simulink model "nn_fuel_control_4_10"  (R2021a)
settings: Solver=ode15s  StartTime=0.0  StopTime=T  MaxStep=.01  RelTol=1e-3
undefined symbols (not defined in the file): AF_sensor_tol, fault_time, fuel_inj_tol, kappa_tol, MAF_sensor_tol, pump_tol, tau_ww_tol
libraries: neural x46
(part 2 of 2)

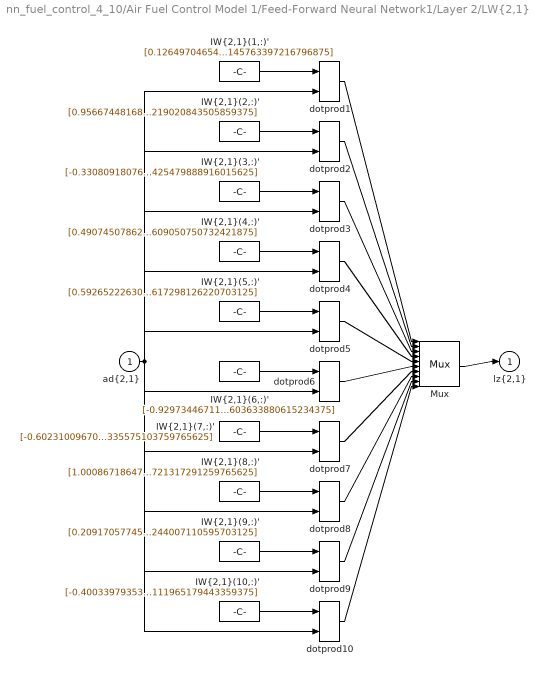
== system nn_fuel_control_4_10/Air Fuel Control Model 1/Feed-Forward Neural Network1/Layer 2/LW{2,1} ==
  "ad{2,1}" : Inport  PortDimensions=10
      mask Display: e = 0.06;c1 = [120 230 180]/255;c2 = ([120 230 180]+0)/(256+128);c3 = ([120 230 180]+128)/(256+128);patch([0 1 1 0],[0 0 1 1],c1);patch([0 1 1 1-e 1-e 0+e],[0 0 1 1-e 0+e 0+e],c2);patch([0 0 1 1-e 0+e 0+e],[0 1 1 1-e 1-e 0+e],c3);plot([0 1 1 0 0],[0 0 1 1 0]);
  "IW{2,1}(1,:)'" : Constant  Value=[0.126497046544859215178036038196296431124210357666015625;0.75221409398679295321699100895784795284271240234375;-0.1950995321727321540894450890846201218664646148681640625;-0.76593928444443459824242381728254258632659912109375;0.06664328726876174446847045373942819423973560333251953125;-0.21742718572034547275251270548324100673198699951171875;1.0030759253859538038256005165749229490756988525390625;-0.7869649700269818470843574687023647129535675048828125;0.556124501951611449612755677662789821624755859375;-0.52293583386677500168815413417178206145763397216796875]
      mask Display: e = 0.06;c1 = [120 150 230]/255;c2 = ([120 150 230]+0)/383;c3 = ([120 150 230]+128)/383;patch([0 1 1 0],[0 0 1 1],c1);patch([0 1 1 1-e 1-e 0+e],[0 0 1 1-e 0+e 0+e],c2);patch([0 0 1 1-e 0+e 0+e],[0 1 1 1-e 1-e 0+e],c3);plot([0 1 1 0 0],[0 0 1 1 0]);disp('weights');
  "IW{2,1}(10,:)'" : Constant  Value=[-0.4003397935387604800183680708869360387325286865234375;-0.9760537487034819381648276248597539961338043212890625;-0.661362482630752257506401292630471289157867431640625;-0.5845508787619853041661599490907974541187286376953125;0.7079823054105311985750859093968756496906280517578125;0.87748572874551289402234033332206308841705322265625;-0.530069953204840516036711051128804683685302734375;-0.848837519709181531624153649318031966686248779296875;-0.9175382615241487460622238359064795076847076416015625;0.27264837844771871999682844034396111965179443359375]
      mask Display: e = 0.06;c1 = [120 150 230]/255;c2 = ([120 150 230]+0)/383;c3 = ([120 150 230]+128)/383;patch([0 1 1 0],[0 0 1 1],c1);patch([0 1 1 1-e 1-e 0+e],[0 0 1 1-e 0+e 0+e],c2);patch([0 0 1 1-e 0+e 0+e],[0 1 1 1-e 1-e 0+e],c3);plot([0 1 1 0 0],[0 0 1 1 0]);disp('weights');
  "IW{2,1}(2,:)'" : Constant  Value=[0.95667448168226798532742805036832578480243682861328125;0.85004275325366618343281288616708479821681976318359375;0.359542314700540099892123180325143039226531982421875;-0.6107936641860096660394674472627229988574981689453125;-0.031298787731731524119904719327678321860730648040771484375;-0.52979378096300411282726372519391588866710662841796875;-0.567955949619257438598651788197457790374755859375;-0.12292161961932319969026394801403512246906757354736328125;0.236880433739087070676987423212267458438873291015625;-0.50914689409082070081780102555057965219020843505859375]
      mask Display: e = 0.06;c1 = [120 150 230]/255;c2 = ([120 150 230]+0)/383;c3 = ([120 150 230]+128)/383;patch([0 1 1 0],[0 0 1 1],c1);patch([0 1 1 1-e 1-e 0+e],[0 0 1 1-e 0+e 0+e],c2);patch([0 0 1 1-e 0+e 0+e],[0 1 1 1-e 1-e 0+e],c3);plot([0 1 1 0 0],[0 0 1 1 0]);disp('weights');
  "IW{2,1}(3,:)'" : Constant  Value=[-0.33080918076060328303356072865426540374755859375;-0.91079242740214727547254369710572063922882080078125;-0.7216409660489764288371361544704996049404144287109375;0.40560109332833160777909142780117690563201904296875;0.7487410521856288081465891082189045846462249755859375;-0.1792937276454249495571957595529966056346893310546875;-0.7489244995021773210197579828673042356967926025390625;-0.950832663107312736627818594570271670818328857421875;-0.98403189361767484655274529359303414821624755859375;-0.594933336252129407739630551077425479888916015625]
      mask Display: e = 0.06;c1 = [120 150 230]/255;c2 = ([120 150 230]+0)/383;c3 = ([120 150 230]+128)/383;patch([0 1 1 0],[0 0 1 1],c1);patch([0 1 1 1-e 1-e 0+e],[0 0 1 1-e 0+e 0+e],c2);patch([0 0 1 1-e 0+e 0+e],[0 1 1 1-e 1-e 0+e],c3);plot([0 1 1 0 0],[0 0 1 1 0]);disp('weights');
  "IW{2,1}(4,:)'" : Constant  Value=[0.490745078629539699388573126270784996449947357177734375;0.669675741776368571578359478735364973545074462890625;-0.7389705859394559706032623580540530383586883544921875;-0.32518846889059016547207647818140685558319091796875;0.7292180816896500772372746723704040050506591796875;0.40551505484997385497791810848866589367389678955078125;-0.8624031920599921630099515823530964553356170654296875;0.406935627679185174532250357515295036137104034423828125;0.82694047359766609250897317906492389738559722900390625;-0.828463743887304371327218177611939609050750732421875]
      mask Display: e = 0.06;c1 = [120 150 230]/255;c2 = ([120 150 230]+0)/383;c3 = ([120 150 230]+128)/383;patch([0 1 1 0],[0 0 1 1],c1);patch([0 1 1 1-e 1-e 0+e],[0 0 1 1-e 0+e 0+e],c2);patch([0 0 1 1-e 0+e 0+e],[0 1 1 1-e 1-e 0+e],c3);plot([0 1 1 0 0],[0 0 1 1 0]);disp('weights');
  "IW{2,1}(5,:)'" : Constant  Value=[0.59265222630545533188950457770260982215404510498046875;0.6513005697610807498421081618289463222026824951171875;0.832729947816391646853162455954588949680328369140625;-0.499949414926917246049242748995311558246612548828125;0.15275099522523305495269596576690673828125;-0.2200642403627948995303853507721214555203914642333984375;0.29279576118233363590803719489485956728458404541015625;0.967351346440282977567903799354098737239837646484375;0.4551810898529715654348137832130305469036102294921875;-0.19101879400775001460743851566803641617298126220703125]
      mask Display: e = 0.06;c1 = [120 150 230]/255;c2 = ([120 150 230]+0)/383;c3 = ([120 150 230]+128)/383;patch([0 1 1 0],[0 0 1 1],c1);patch([0 1 1 1-e 1-e 0+e],[0 0 1 1-e 0+e 0+e],c2);patch([0 0 1 1-e 0+e 0+e],[0 1 1 1-e 1-e 0+e],c3);plot([0 1 1 0 0],[0 0 1 1 0]);disp('weights');
  "IW{2,1}(6,:)'" : Constant  Value=[-0.929734467111477780321138197905384004116058349609375;-0.20633861665115471595299823093228042125701904296875;0.243861218275130742227929658838547766208648681640625;-0.1569894136270153506274027677136473357677459716796875;-0.1436763750970591058120362504268996417522430419921875;-0.721299534939905395702908208477310836315155029296875;-0.8723462156088059860081784790963865816593170166015625;-0.7906932906879029498981026335968635976314544677734375;-0.2135932946365211027028863099985755980014801025390625;0.625957171841073911622288505895994603633880615234375]
      mask Display: e = 0.06;c1 = [120 150 230]/255;c2 = ([120 150 230]+0)/383;c3 = ([120 150 230]+128)/383;patch([0 1 1 0],[0 0 1 1],c1);patch([0 1 1 1-e 1-e 0+e],[0 0 1 1-e 0+e 0+e],c2);patch([0 0 1 1-e 0+e 0+e],[0 1 1 1-e 1-e 0+e],c3);plot([0 1 1 0 0],[0 0 1 1 0]);disp('weights');
  "IW{2,1}(7,:)'" : Constant  Value=[-0.602310096703943198548358850530348718166351318359375;0.73376329364989967274368609650991857051849365234375;0.95498454377033947793051993357948958873748779296875;0.9141420095755534713788392764399759471416473388671875;-0.99757823216680474587292337673716247081756591796875;0.388190532974689528344924838165752589702606201171875;0.232893122124527618410638751811347901821136474609375;0.4600844221479103435257229648414067924022674560546875;-0.4005592463439544559378191479481756687164306640625;-0.4404459192897596242488589268759824335575103759765625]
      mask Display: e = 0.06;c1 = [120 150 230]/255;c2 = ([120 150 230]+0)/383;c3 = ([120 150 230]+128)/383;patch([0 1 1 0],[0 0 1 1],c1);patch([0 1 1 1-e 1-e 0+e],[0 0 1 1-e 0+e 0+e],c2);patch([0 0 1 1-e 0+e 0+e],[0 1 1 1-e 1-e 0+e],c3);plot([0 1 1 0 0],[0 0 1 1 0]);disp('weights');
  "IW{2,1}(8,:)'" : Constant  Value=[1.0008671864742602064524135130341164767742156982421875;0.627994547262577640367453568615019321441650390625;-0.4388968675581679246278099526534788310527801513671875;-0.663554034333136311119005767977796494960784912109375;-0.40036111281525454952401332775480113923549652099609375;0.53464556671534901877151924054487608373165130615234375;-0.48995700829802946163482602059957571327686309814453125;0.93419460342121940499282573000527918338775634765625;0.60615497083046887549784287330112420022487640380859375;0.88538726723761718151450850200490094721317291259765625]
      mask Display: e = 0.06;c1 = [120 150 230]/255;c2 = ([120 150 230]+0)/383;c3 = ([120 150 230]+128)/383;patch([0 1 1 0],[0 0 1 1],c1);patch([0 1 1 1-e 1-e 0+e],[0 0 1 1-e 0+e 0+e],c2);patch([0 0 1 1-e 0+e 0+e],[0 1 1 1-e 1-e 0+e],c3);plot([0 1 1 0 0],[0 0 1 1 0]);disp('weights');
  "IW{2,1}(9,:)'" : Constant  Value=[0.2091705774532304218382705585099756717681884765625;-0.80315186566978546967021657110308296978473663330078125;-0.64306646193011574030862220752169378101825714111328125;0.2163986745118722243574893582263030111789703369140625;0.9081691422474353903027122214552946388721466064453125;-0.144285445670728817990635661772103048861026763916015625;-0.82048635195377761508694902659044601023197174072265625;-0.09813172413988389963801495241568773053586483001708984375;0.2346797496115521630688505183570669032633304595947265625;0.7056863914651156921564734147978015244007110595703125]
      mask Display: e = 0.06;c1 = [120 150 230]/255;c2 = ([120 150 230]+0)/383;c3 = ([120 150 230]+128)/383;patch([0 1 1 0],[0 0 1 1],c1);patch([0 1 1 1-e 1-e 0+e],[0 0 1 1-e 0+e 0+e],c2);patch([0 0 1 1-e 0+e 0+e],[0 1 1 1-e 1-e 0+e],c3);plot([0 1 1 0 0],[0 0 1 1 0]);disp('weights');
  Mux : Mux  Inputs=10
      mask Display: e = 0.06;c1 = [120 150 230]/255;c2 = ([120 150 230]+0)/383;c3 = ([120 150 230]+128)/383;patch([0 1 1 0],[0 0 1 1],c1);patch([0 1 1 1-e 1-e 0+e],[0 0 1 1-e 0+e 0+e],c2);patch([0 0 1 1-e 0+e 0+e],[0 1 1 1-e 1-e 0+e],c3);plot([0 1 1 0 0],[0 0 1 1 0]);disp('Mux');
  dotprod{1..10} (10 alike) : neural/Weight Functions/dotprod
  "lz{2,1}" : Outport
      mask Display: e = 0.06;c1 = [120 230 180]/255;c2 = ([120 230 180]+0)/(256+128);c3 = ([120 230 180]+128)/(256+128);patch([0 1 1 0],[0 0 1 1],c1);patch([0 1 1 1-e 1-e 0+e],[0 0 1 1-e 0+e 0+e],c2);patch([0 0 1 1-e 0+e 0+e],[0 1 1 1-e 1-e 0+e],c3);plot([0 1 1 0 0],[0 0 1 1 0]);
  wires:
  "IW{2,1}(1,:)'"/1 -> dotprod1/1
  "ad{2,1}"/1 -> dotprod1/2, dotprod2/2, dotprod3/2, dotprod4/2, dotprod5/2, dotprod6/2, dotprod7/2, dotprod8/2, dotprod9/2, dotprod10/2
  dotprod1/1 -> Mux/1
  "IW{2,1}(2,:)'"/1 -> dotprod2/1
  dotprod2/1 -> Mux/2
  "IW{2,1}(3,:)'"/1 -> dotprod3/1
  dotprod3/1 -> Mux/3
  "IW{2,1}(4,:)'"/1 -> dotprod4/1
  dotprod4/1 -> Mux/4
  "IW{2,1}(5,:)'"/1 -> dotprod5/1
  dotprod5/1 -> Mux/5
  "IW{2,1}(6,:)'"/1 -> dotprod6/1
  dotprod6/1 -> Mux/6
  "IW{2,1}(7,:)'"/1 -> dotprod7/1
  dotprod7/1 -> Mux/7
  "IW{2,1}(8,:)'"/1 -> dotprod8/1
  dotprod8/1 -> Mux/8
  "IW{2,1}(9,:)'"/1 -> dotprod9/1
  dotprod9/1 -> Mux/9
  "IW{2,1}(10,:)'"/1 -> dotprod10/1
  dotprod10/1 -> Mux/10
  Mux/1 -> "lz{2,1}"/1

== system nn_fuel_control_4_10/Air Fuel Control Model 1/Feed-Forward Neural Network1/Layer 3/Delays 1 ==
  "p{3}" : Inport  PortDimensions=10
      mask Display: e = 0.06;c1 = [120 230 180]/255;c2 = ([120 230 180]+0)/(256+128);c3 = ([120 230 180]+128)/(256+128);patch([0 1 1 0],[0 0 1 1],c1);patch([0 1 1 1-e 1-e 0+e],[0 0 1 1-e 0+e 0+e],c2);patch([0 0 1 1-e 0+e 0+e],[0 1 1 1-e 1-e 0+e],c3);plot([0 1 1 0 0],[0 0 1 1 0]);
  mux : Mux  Inputs=1
      mask Display: e = 0.06;c1 = [120 150 230]/255;c2 = ([120 150 230]+0)/383;c3 = ([120 150 230]+128)/383;patch([0 1 1 0],[0 0 1 1],c1);patch([0 1 1 1-e 1-e 0+e],[0 0 1 1-e 0+e 0+e],c2);patch([0 0 1 1-e 0+e 0+e],[0 1 1 1-e 1-e 0+e],c3);plot([0 1 1 0 0],[0 0 1 1 0]);disp('Mux')
  "pd{3,2}" : Outport
      mask Display: e = 0.06;c1 = [120 230 180]/255;c2 = ([120 230 180]+0)/(256+128);c3 = ([120 230 180]+128)/(256+128);patch([0 1 1 0],[0 0 1 1],c1);patch([0 1 1 1-e 1-e 0+e],[0 0 1 1-e 0+e 0+e],c2);patch([0 0 1 1-e 0+e 0+e],[0 1 1 1-e 1-e 0+e],c3);plot([0 1 1 0 0],[0 0 1 1 0]);
  wires:
  "p{3}"/1 -> mux/1
  mux/1 -> "pd{3,2}"/1

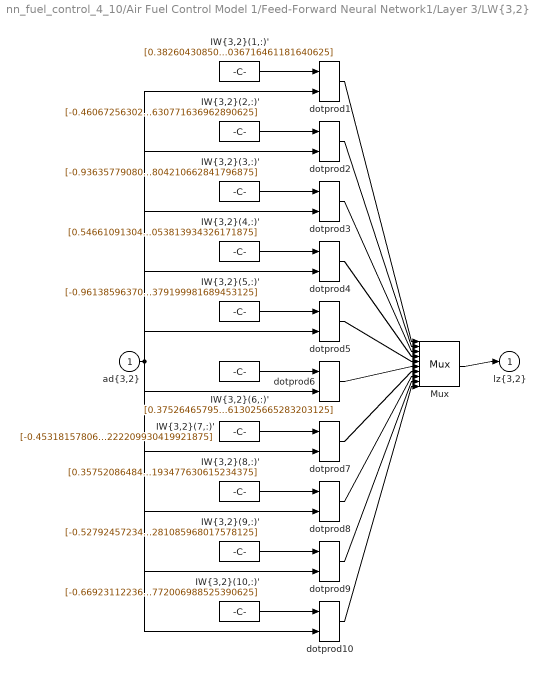
== system nn_fuel_control_4_10/Air Fuel Control Model 1/Feed-Forward Neural Network1/Layer 3/LW{3,2} ==
  "ad{3,2}" : Inport  PortDimensions=10
      mask Display: e = 0.06;c1 = [120 230 180]/255;c2 = ([120 230 180]+0)/(256+128);c3 = ([120 230 180]+128)/(256+128);patch([0 1 1 0],[0 0 1 1],c1);patch([0 1 1 1-e 1-e 0+e],[0 0 1 1-e 0+e 0+e],c2);patch([0 0 1 1-e 0+e 0+e],[0 1 1 1-e 1-e 0+e],c3);plot([0 1 1 0 0],[0 0 1 1 0]);
  "IW{3,2}(1,:)'" : Constant  Value=[0.38260430850073368080899172127828933298587799072265625;0.13642733469780454758080168176093138754367828369140625;-0.095958036144256908528404892422258853912353515625;0.36174155693469034478226831197389401495456695556640625;0.8350602437937642008591865305788815021514892578125;0.3251084275911748644460885770968161523342132568359375;0.3030576797765258678651889567845501005649566650390625;0.499262400095795533250253583901212550699710845947265625;-0.50310955428479786633033654652535915374755859375;0.488601647793304838529593325802125036716461181640625]
      mask Display: e = 0.06;c1 = [120 150 230]/255;c2 = ([120 150 230]+0)/383;c3 = ([120 150 230]+128)/383;patch([0 1 1 0],[0 0 1 1],c1);patch([0 1 1 1-e 1-e 0+e],[0 0 1 1-e 0+e 0+e],c2);patch([0 0 1 1-e 0+e 0+e],[0 1 1 1-e 1-e 0+e],c3);plot([0 1 1 0 0],[0 0 1 1 0]);disp('weights');
  "IW{3,2}(10,:)'" : Constant  Value=[-0.6692311223638414130476803620695136487483978271484375;-0.6645229148138138697277099709026515483856201171875;0.158812055333411361601747557870112359523773193359375;-0.3401238183278600946124470283393748104572296142578125;-0.600266633534465743338159882114268839359283447265625;0.679217684825130785242208730778656899929046630859375;-0.8769909030569105201635693447315134108066558837890625;-0.804965185234801428038053927593864500522613525390625;-0.2273698401426849091677695469115860760211944580078125;-0.7084831043194095290260747788124717772006988525390625]
      mask Display: e = 0.06;c1 = [120 150 230]/255;c2 = ([120 150 230]+0)/383;c3 = ([120 150 230]+128)/383;patch([0 1 1 0],[0 0 1 1],c1);patch([0 1 1 1-e 1-e 0+e],[0 0 1 1-e 0+e 0+e],c2);patch([0 0 1 1-e 0+e 0+e],[0 1 1 1-e 1-e 0+e],c3);plot([0 1 1 0 0],[0 0 1 1 0]);disp('weights');
  "IW{3,2}(2,:)'" : Constant  Value=[-0.4606725630226671253097947555943392217159271240234375;-0.5148795137688690903843280466389842331409454345703125;-0.6540856842614874988584006132441572844982147216796875;-0.3533807951762197863132541897357441484928131103515625;0.02258533808582097179851189139299094676971435546875;0.0214007259205357680542647358379326760768890380859375;-0.693474210329056983681539350072853267192840576171875;-0.232900610784799066976802350836805999279022216796875;-0.77176012166602259156888976576738059520721435546875;0.8126773180502144811043763183988630771636962890625]
      mask Display: e = 0.06;c1 = [120 150 230]/255;c2 = ([120 150 230]+0)/383;c3 = ([120 150 230]+128)/383;patch([0 1 1 0],[0 0 1 1],c1);patch([0 1 1 1-e 1-e 0+e],[0 0 1 1-e 0+e 0+e],c2);patch([0 0 1 1-e 0+e 0+e],[0 1 1 1-e 1-e 0+e],c3);plot([0 1 1 0 0],[0 0 1 1 0]);disp('weights');
  "IW{3,2}(3,:)'" : Constant  Value=[-0.9363577908057532095398300953092984855175018310546875;-0.5103928923824501140416032285429537296295166015625;-0.1517970185541290817354820319451391696929931640625;-0.685862683587971755372336701839230954647064208984375;-0.209173333676665240687952973530627787113189697265625;0.9361149605558534148030958021990954875946044921875;-0.198203550068528411287616108893416821956634521484375;-0.15049364937842835132641994277946650981903076171875;-0.11084201640954116641069049364887177944183349609375;-0.797224114677578921117628851789049804210662841796875]
      mask Display: e = 0.06;c1 = [120 150 230]/255;c2 = ([120 150 230]+0)/383;c3 = ([120 150 230]+128)/383;patch([0 1 1 0],[0 0 1 1],c1);patch([0 1 1 1-e 1-e 0+e],[0 0 1 1-e 0+e 0+e],c2);patch([0 0 1 1-e 0+e 0+e],[0 1 1 1-e 1-e 0+e],c3);plot([0 1 1 0 0],[0 0 1 1 0]);disp('weights');
  "IW{3,2}(4,:)'" : Constant  Value=[0.5466109130413598915509965081582777202129364013671875;-0.3733089710438990405094727975665591657161712646484375;0.50422650592085727083713209140114486217498779296875;-0.33519853633565421802131822914816439151763916015625;-0.932887593629181832710628441418521106243133544921875;0.8554786036908088586727672009146772325038909912109375;-0.6750587219550965301095857284963130950927734375;-0.2438384706562761738979361325618810951709747314453125;0.99084902965801280316782140289433300495147705078125;-0.1548693654204285063968882241169922053813934326171875]
      mask Display: e = 0.06;c1 = [120 150 230]/255;c2 = ([120 150 230]+0)/383;c3 = ([120 150 230]+128)/383;patch([0 1 1 0],[0 0 1 1],c1);patch([0 1 1 1-e 1-e 0+e],[0 0 1 1-e 0+e 0+e],c2);patch([0 0 1 1-e 0+e 0+e],[0 1 1 1-e 1-e 0+e],c3);plot([0 1 1 0 0],[0 0 1 1 0]);disp('weights');
  "IW{3,2}(5,:)'" : Constant  Value=[-0.961385963701682388915514820837415754795074462890625;-0.3054993719950829245135537348687648773193359375;0.7823990784192005332187136446009390056133270263671875;0.2401319377577852964833482474205084145069122314453125;-0.9064006789198890690073540099547244608402252197265625;-0.2655667047827423576933369986363686621189117431640625;-0.289044106223085517370918751112185418605804443359375;0.196156308789054545371755011728964745998382568359375;-0.449488780935833887042463175021111965179443359375;0.93688112513218602117603950318880379199981689453125]
      mask Display: e = 0.06;c1 = [120 150 230]/255;c2 = ([120 150 230]+0)/383;c3 = ([120 150 230]+128)/383;patch([0 1 1 0],[0 0 1 1],c1);patch([0 1 1 1-e 1-e 0+e],[0 0 1 1-e 0+e 0+e],c2);patch([0 0 1 1-e 0+e 0+e],[0 1 1 1-e 1-e 0+e],c3);plot([0 1 1 0 0],[0 0 1 1 0]);disp('weights');
  "IW{3,2}(6,:)'" : Constant  Value=[0.375264657950043878376078509973012842237949371337890625;0.678663362574325912390804660390131175518035888671875;-0.0154345293262334593009654781781136989593505859375;-0.88870813588056651877167269049095921218395233154296875;0.375156911910723145364698893899912945926189422607421875;0.509254696911920490265401895157992839813232421875;0.4095385198210583777012061545974574983119964599609375;-0.2131265080635856012936102388266590423882007598876953125;0.80056353697317916839892859570682048797607421875;0.728746013054529573338413683813996613025665283203125]
      mask Display: e = 0.06;c1 = [120 150 230]/255;c2 = ([120 150 230]+0)/383;c3 = ([120 150 230]+128)/383;patch([0 1 1 0],[0 0 1 1],c1);patch([0 1 1 1-e 1-e 0+e],[0 0 1 1-e 0+e 0+e],c2);patch([0 0 1 1-e 0+e 0+e],[0 1 1 1-e 1-e 0+e],c3);plot([0 1 1 0 0],[0 0 1 1 0]);disp('weights');
  "IW{3,2}(7,:)'" : Constant  Value=[-0.453181578066854051645151457705651409924030303955078125;-0.669208524680863892086790656321682035923004150390625;0.46056123971567597408238725620321929454803466796875;0.183054237740345848717282706275000236928462982177734375;0.98965338045430162328131018512067385017871856689453125;0.4481354634721761431848108259146101772785186767578125;-0.842689642823334583709993239608593285083770751953125;0.1455283589027605850585445068645640276372432708740234375;-0.91386113632724585986721876906813122332096099853515625;0.26811149082483165528856261516921222209930419921875]
      mask Display: e = 0.06;c1 = [120 150 230]/255;c2 = ([120 150 230]+0)/383;c3 = ([120 150 230]+128)/383;patch([0 1 1 0],[0 0 1 1],c1);patch([0 1 1 1-e 1-e 0+e],[0 0 1 1-e 0+e 0+e],c2);patch([0 0 1 1-e 0+e 0+e],[0 1 1 1-e 1-e 0+e],c3);plot([0 1 1 0 0],[0 0 1 1 0]);disp('weights');
  "IW{3,2}(8,:)'" : Constant  Value=[0.357520864843551777756402998420526273548603057861328125;0.12432599689534802600565654984166030772030353546142578125;-0.467357290617872234150809163111262023448944091796875;-0.1581695296183729115835348011387395672500133514404296875;0.96924978167168018838850684915087185800075531005859375;0.074141279121479275460160351940430700778961181640625;-0.49420729356245107766198998433537781238555908203125;-0.374908193137290235430469920174800790846347808837890625;0.639944783647838022488940623588860034942626953125;-0.24179273998143369084345977171324193477630615234375]
      mask Display: e = 0.06;c1 = [120 150 230]/255;c2 = ([120 150 230]+0)/383;c3 = ([120 150 230]+128)/383;patch([0 1 1 0],[0 0 1 1],c1);patch([0 1 1 1-e 1-e 0+e],[0 0 1 1-e 0+e 0+e],c2);patch([0 0 1 1-e 0+e 0+e],[0 1 1 1-e 1-e 0+e],c3);plot([0 1 1 0 0],[0 0 1 1 0]);disp('weights');
  "IW{3,2}(9,:)'" : Constant  Value=[-0.52792457234601830595721594363567419350147247314453125;-0.6946178384078256495826053651398979127407073974609375;-0.7549504683775685176527758812881074845790863037109375;0.3374971400659443343528209879877977073192596435546875;0.371679393645964084580413100411533378064632415771484375;-0.190977195230001672854314165306277573108673095703125;0.009978535841423497032565137487836182117462158203125;0.94404664177656705259522595952148549258708953857421875;0.0088254457175579170691293029449298046529293060302734375;0.781339013056147724256561559741385281085968017578125]
      mask Display: e = 0.06;c1 = [120 150 230]/255;c2 = ([120 150 230]+0)/383;c3 = ([120 150 230]+128)/383;patch([0 1 1 0],[0 0 1 1],c1);patch([0 1 1 1-e 1-e 0+e],[0 0 1 1-e 0+e 0+e],c2);patch([0 0 1 1-e 0+e 0+e],[0 1 1 1-e 1-e 0+e],c3);plot([0 1 1 0 0],[0 0 1 1 0]);disp('weights');
  Mux : Mux  Inputs=10
      mask Display: e = 0.06;c1 = [120 150 230]/255;c2 = ([120 150 230]+0)/383;c3 = ([120 150 230]+128)/383;patch([0 1 1 0],[0 0 1 1],c1);patch([0 1 1 1-e 1-e 0+e],[0 0 1 1-e 0+e 0+e],c2);patch([0 0 1 1-e 0+e 0+e],[0 1 1 1-e 1-e 0+e],c3);plot([0 1 1 0 0],[0 0 1 1 0]);disp('Mux');
  dotprod{1..10} (10 alike) : neural/Weight Functions/dotprod
  "lz{3,2}" : Outport
      mask Display: e = 0.06;c1 = [120 230 180]/255;c2 = ([120 230 180]+0)/(256+128);c3 = ([120 230 180]+128)/(256+128);patch([0 1 1 0],[0 0 1 1],c1);patch([0 1 1 1-e 1-e 0+e],[0 0 1 1-e 0+e 0+e],c2);patch([0 0 1 1-e 0+e 0+e],[0 1 1 1-e 1-e 0+e],c3);plot([0 1 1 0 0],[0 0 1 1 0]);
  wires:
  "IW{3,2}(1,:)'"/1 -> dotprod1/1
  "ad{3,2}"/1 -> dotprod1/2, dotprod2/2, dotprod3/2, dotprod4/2, dotprod5/2, dotprod6/2, dotprod7/2, dotprod8/2, dotprod9/2, dotprod10/2
  dotprod1/1 -> Mux/1
  "IW{3,2}(2,:)'"/1 -> dotprod2/1
  dotprod2/1 -> Mux/2
  "IW{3,2}(3,:)'"/1 -> dotprod3/1
  dotprod3/1 -> Mux/3
  "IW{3,2}(4,:)'"/1 -> dotprod4/1
  dotprod4/1 -> Mux/4
  "IW{3,2}(5,:)'"/1 -> dotprod5/1
  dotprod5/1 -> Mux/5
  "IW{3,2}(6,:)'"/1 -> dotprod6/1
  dotprod6/1 -> Mux/6
  "IW{3,2}(7,:)'"/1 -> dotprod7/1
  dotprod7/1 -> Mux/7
  "IW{3,2}(8,:)'"/1 -> dotprod8/1
  dotprod8/1 -> Mux/8
  "IW{3,2}(9,:)'"/1 -> dotprod9/1
  dotprod9/1 -> Mux/9
  "IW{3,2}(10,:)'"/1 -> dotprod10/1
  dotprod10/1 -> Mux/10
  Mux/1 -> "lz{3,2}"/1

== system nn_fuel_control_4_10/Air Fuel Control Model 1/Feed-Forward Neural Network1/Layer 4/Delays 1 ==
  "p{4}" : Inport  PortDimensions=10
      mask Display: e = 0.06;c1 = [120 230 180]/255;c2 = ([120 230 180]+0)/(256+128);c3 = ([120 230 180]+128)/(256+128);patch([0 1 1 0],[0 0 1 1],c1);patch([0 1 1 1-e 1-e 0+e],[0 0 1 1-e 0+e 0+e],c2);patch([0 0 1 1-e 0+e 0+e],[0 1 1 1-e 1-e 0+e],c3);plot([0 1 1 0 0],[0 0 1 1 0]);
  mux : Mux  Inputs=1
      mask Display: e = 0.06;c1 = [120 150 230]/255;c2 = ([120 150 230]+0)/383;c3 = ([120 150 230]+128)/383;patch([0 1 1 0],[0 0 1 1],c1);patch([0 1 1 1-e 1-e 0+e],[0 0 1 1-e 0+e 0+e],c2);patch([0 0 1 1-e 0+e 0+e],[0 1 1 1-e 1-e 0+e],c3);plot([0 1 1 0 0],[0 0 1 1 0]);disp('Mux')
  "pd{4,3}" : Outport
      mask Display: e = 0.06;c1 = [120 230 180]/255;c2 = ([120 230 180]+0)/(256+128);c3 = ([120 230 180]+128)/(256+128);patch([0 1 1 0],[0 0 1 1],c1);patch([0 1 1 1-e 1-e 0+e],[0 0 1 1-e 0+e 0+e],c2);patch([0 0 1 1-e 0+e 0+e],[0 1 1 1-e 1-e 0+e],c3);plot([0 1 1 0 0],[0 0 1 1 0]);
  wires:
  "p{4}"/1 -> mux/1
  mux/1 -> "pd{4,3}"/1

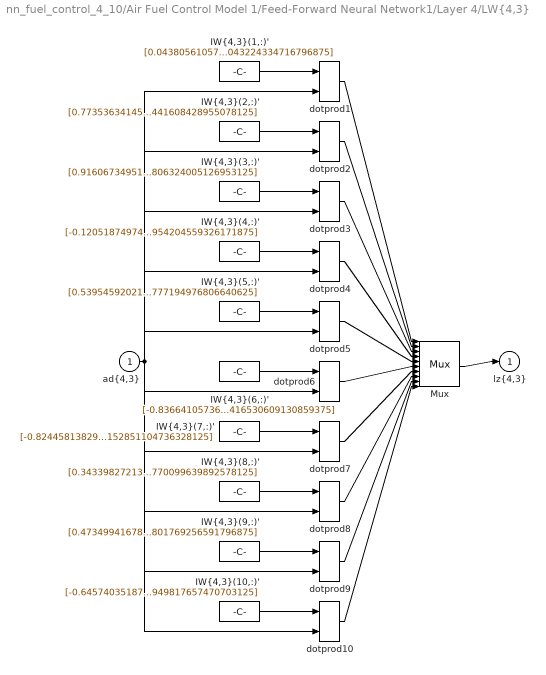
== system nn_fuel_control_4_10/Air Fuel Control Model 1/Feed-Forward Neural Network1/Layer 4/LW{4,3} ==
  "ad{4,3}" : Inport  PortDimensions=10
      mask Display: e = 0.06;c1 = [120 230 180]/255;c2 = ([120 230 180]+0)/(256+128);c3 = ([120 230 180]+128)/(256+128);patch([0 1 1 0],[0 0 1 1],c1);patch([0 1 1 1-e 1-e 0+e],[0 0 1 1-e 0+e 0+e],c2);patch([0 0 1 1-e 0+e 0+e],[0 1 1 1-e 1-e 0+e],c3);plot([0 1 1 0 0],[0 0 1 1 0]);
  "IW{4,3}(1,:)'" : Constant  Value=[0.04380561057782660083770309711326262913644313812255859375;0.2036798576520684189716803302871994674205780029296875;0.724715622228626177303567601484246551990509033203125;-0.07546146495840755363815333112142980098724365234375;0.2490632762087379159510192039306275546550750732421875;-0.0213081585611721753548142288536837440915405750274658203125;0.9435288967462220899307112631504423916339874267578125;0.307607917622672533131122918348410166800022125244140625;-0.3731209230014951305776094159227795898914337158203125;-0.943713327778044952509617360192351043224334716796875]
      mask Display: e = 0.06;c1 = [120 150 230]/255;c2 = ([120 150 230]+0)/383;c3 = ([120 150 230]+128)/383;patch([0 1 1 0],[0 0 1 1],c1);patch([0 1 1 1-e 1-e 0+e],[0 0 1 1-e 0+e 0+e],c2);patch([0 0 1 1-e 0+e 0+e],[0 1 1 1-e 1-e 0+e],c3);plot([0 1 1 0 0],[0 0 1 1 0]);disp('weights');
  "IW{4,3}(10,:)'" : Constant  Value=[-0.6457403518731854585865903572994284331798553466796875;0.4997551457461468782383917641709558665752410888671875;0.7213603635096041966079383200849406421184539794921875;0.0999357244721374993190465829684399068355560302734375;-0.8327561514013936960765249750693328678607940673828125;-0.33598059057347828826323166140355169773101806640625;0.757253462340730987278902830439619719982147216796875;0.6081551380829661734850333232316188514232635498046875;-0.9090301417166930519897505291737616062164306640625;-0.3353810826422229940391162017476744949817657470703125]
      mask Display: e = 0.06;c1 = [120 150 230]/255;c2 = ([120 150 230]+0)/383;c3 = ([120 150 230]+128)/383;patch([0 1 1 0],[0 0 1 1],c1);patch([0 1 1 1-e 1-e 0+e],[0 0 1 1-e 0+e 0+e],c2);patch([0 0 1 1-e 0+e 0+e],[0 1 1 1-e 1-e 0+e],c3);plot([0 1 1 0 0],[0 0 1 1 0]);disp('weights');
  "IW{4,3}(2,:)'" : Constant  Value=[0.77353634145463889826288550466415472328662872314453125;-0.059590631807953542420364101417362689971923828125;-0.3447007246868241114867714713909663259983062744140625;0.603165314444659816928151485626585781574249267578125;0.0154626781197035878534506991854868829250335693359375;0.1036427108369364358253505997708998620510101318359375;-0.1907772976114223972832206754901562817394733428955078125;-0.438318463902227561934665800436050631105899810791015625;0.90910247482883921321672460180707275867462158203125;0.0420546394594367711761151440441608428955078125]
      mask Display: e = 0.06;c1 = [120 150 230]/255;c2 = ([120 150 230]+0)/383;c3 = ([120 150 230]+128)/383;patch([0 1 1 0],[0 0 1 1],c1);patch([0 1 1 1-e 1-e 0+e],[0 0 1 1-e 0+e 0+e],c2);patch([0 0 1 1-e 0+e 0+e],[0 1 1 1-e 1-e 0+e],c3);plot([0 1 1 0 0],[0 0 1 1 0]);disp('weights');
  "IW{4,3}(3,:)'" : Constant  Value=[0.91606734951941837241662369706318713724613189697265625;-0.938738128790599812845130145433358848094940185546875;0.0537253627939779931921293609775602817535400390625;-0.1279369897601962957622845351579599082469940185546875;0.130753279242124431647198434802703559398651123046875;-0.673870637978049469296593088074587285518646240234375;0.294053993085480580571555719870957545936107635498046875;-0.65102166919441206704988189812866039574146270751953125;0.5336923860716911161006237307447008788585662841796875;-0.3863597356441463848142348069814033806324005126953125]
      mask Display: e = 0.06;c1 = [120 150 230]/255;c2 = ([120 150 230]+0)/383;c3 = ([120 150 230]+128)/383;patch([0 1 1 0],[0 0 1 1],c1);patch([0 1 1 1-e 1-e 0+e],[0 0 1 1-e 0+e 0+e],c2);patch([0 0 1 1-e 0+e 0+e],[0 1 1 1-e 1-e 0+e],c3);plot([0 1 1 0 0],[0 0 1 1 0]);disp('weights');
  "IW{4,3}(4,:)'" : Constant  Value=[-0.1205187497489941250705669517628848552703857421875;0.7165426350445331937777382336207665503025054931640625;0.110060707784299438571906648576259613037109375;-0.76515620329558853285334407701157033443450927734375;-0.5257970268697846893957148495246656239032745361328125;-0.430810952527155510694001350202597677707672119140625;0.2731053139965167186886674244306050240993499755859375;-0.330188036439510224084870060323737561702728271484375;-0.84232257109947017426065940526314079761505126953125;-0.3745309139891801475386046149651519954204559326171875]
      mask Display: e = 0.06;c1 = [120 150 230]/255;c2 = ([120 150 230]+0)/383;c3 = ([120 150 230]+128)/383;patch([0 1 1 0],[0 0 1 1],c1);patch([0 1 1 1-e 1-e 0+e],[0 0 1 1-e 0+e 0+e],c2);patch([0 0 1 1-e 0+e 0+e],[0 1 1 1-e 1-e 0+e],c3);plot([0 1 1 0 0],[0 0 1 1 0]);disp('weights');
  "IW{4,3}(5,:)'" : Constant  Value=[0.53954592021344394137116751153371296823024749755859375;-0.06677217914445510160703634028322994709014892578125;0.839828319568382664073169507901184260845184326171875;0.200556834430815289493921227403916418552398681640625;-0.06039996061147601125185246928595006465911865234375;-0.53393408852305146439221061882562935352325439453125;0.474211875557534467962028656984330154955387115478515625;-0.003385968252282259803587205482244826271198689937591552734375;-0.72893206159857160120196795105584897100925445556640625;-0.8994505131360173155741222217329777777194976806640625]
      mask Display: e = 0.06;c1 = [120 150 230]/255;c2 = ([120 150 230]+0)/383;c3 = ([120 150 230]+128)/383;patch([0 1 1 0],[0 0 1 1],c1);patch([0 1 1 1-e 1-e 0+e],[0 0 1 1-e 0+e 0+e],c2);patch([0 0 1 1-e 0+e 0+e],[0 1 1 1-e 1-e 0+e],c3);plot([0 1 1 0 0],[0 0 1 1 0]);disp('weights');
  "IW{4,3}(6,:)'" : Constant  Value=[-0.8366410573609426304386715855798684060573577880859375;0.5102540287171153376988286254345439374446868896484375;-0.3493973365351645821164083827170543372631072998046875;0.5726987712446300893276429633260704576969146728515625;-0.9606605961189151887680282015935517847537994384765625;-0.585216927846402779067602750728838145732879638671875;0.100200761038979013761718306341208517551422119140625;-0.35953610874305841349496404291130602359771728515625;0.041770415595579368783774043549783527851104736328125;0.283702330652841450131518286070786416530609130859375]
      mask Display: e = 0.06;c1 = [120 150 230]/255;c2 = ([120 150 230]+0)/383;c3 = ([120 150 230]+128)/383;patch([0 1 1 0],[0 0 1 1],c1);patch([0 1 1 1-e 1-e 0+e],[0 0 1 1-e 0+e 0+e],c2);patch([0 0 1 1-e 0+e 0+e],[0 1 1 1-e 1-e 0+e],c3);plot([0 1 1 0 0],[0 0 1 1 0]);disp('weights');
  "IW{4,3}(7,:)'" : Constant  Value=[-0.824458138293965969722876252490095794200897216796875;-0.0221833076780486582180174082168377935886383056640625;-0.4369937103415484358492903993465006351470947265625;0.6583205693883871223448522869148291647434234619140625;0.8964769377251602389122808745014481246471405029296875;-0.0562760465050657909813480728189460933208465576171875;0.7222315319057290849968921975232660770416259765625;0.2301246385770283620075815633754245936870574951171875;-0.6619821655820798955716099953860975801944732666015625;-0.1200866117953751643909754420747049152851104736328125]
      mask Display: e = 0.06;c1 = [120 150 230]/255;c2 = ([120 150 230]+0)/383;c3 = ([120 150 230]+128)/383;patch([0 1 1 0],[0 0 1 1],c1);patch([0 1 1 1-e 1-e 0+e],[0 0 1 1-e 0+e 0+e],c2);patch([0 0 1 1-e 0+e 0+e],[0 1 1 1-e 1-e 0+e],c3);plot([0 1 1 0 0],[0 0 1 1 0]);disp('weights');
  "IW{4,3}(8,:)'" : Constant  Value=[0.343398272133736248701296744911815039813518524169921875;-0.6337089092395353784326061941101215779781341552734375;0.48887465014859987633144555729813873767852783203125;-0.2178178229953104949601083717425353825092315673828125;0.59443630053708407245949274511076509952545166015625;-0.1289895229974437340647597238785238005220890045166015625;0.56518987816038912530558491198462434113025665283203125;-0.1367138140467472895434042357010184787213802337646484375;-0.81408274889089560222288355362252332270145416259765625;0.4390019702672340873306211506132967770099639892578125]
      mask Display: e = 0.06;c1 = [120 150 230]/255;c2 = ([120 150 230]+0)/383;c3 = ([120 150 230]+128)/383;patch([0 1 1 0],[0 0 1 1],c1);patch([0 1 1 1-e 1-e 0+e],[0 0 1 1-e 0+e 0+e],c2);patch([0 0 1 1-e 0+e 0+e],[0 1 1 1-e 1-e 0+e],c3);plot([0 1 1 0 0],[0 0 1 1 0]);disp('weights');
  "IW{4,3}(9,:)'" : Constant  Value=[0.4734994167850550272902410142705775797367095947265625;-0.077061438671368165387320914305746555328369140625;-0.9371027031412431096413229170138947665691375732421875;0.400167362846276741805695564835332334041595458984375;-0.918770511030852166101112743490375578403472900390625;0.6817806863773794301408770479611121118068695068359375;0.8508730110667936941126754391007125377655029296875;-0.475578968917821642836685214206227101385593414306640625;-0.38398083777258751325689445366151630878448486328125;-0.8930784587576265920461082714609801769256591796875]
      mask Display: e = 0.06;c1 = [120 150 230]/255;c2 = ([120 150 230]+0)/383;c3 = ([120 150 230]+128)/383;patch([0 1 1 0],[0 0 1 1],c1);patch([0 1 1 1-e 1-e 0+e],[0 0 1 1-e 0+e 0+e],c2);patch([0 0 1 1-e 0+e 0+e],[0 1 1 1-e 1-e 0+e],c3);plot([0 1 1 0 0],[0 0 1 1 0]);disp('weights');
  Mux : Mux  Inputs=10
      mask Display: e = 0.06;c1 = [120 150 230]/255;c2 = ([120 150 230]+0)/383;c3 = ([120 150 230]+128)/383;patch([0 1 1 0],[0 0 1 1],c1);patch([0 1 1 1-e 1-e 0+e],[0 0 1 1-e 0+e 0+e],c2);patch([0 0 1 1-e 0+e 0+e],[0 1 1 1-e 1-e 0+e],c3);plot([0 1 1 0 0],[0 0 1 1 0]);disp('Mux');
  dotprod{1..10} (10 alike) : neural/Weight Functions/dotprod
  "lz{4,3}" : Outport
      mask Display: e = 0.06;c1 = [120 230 180]/255;c2 = ([120 230 180]+0)/(256+128);c3 = ([120 230 180]+128)/(256+128);patch([0 1 1 0],[0 0 1 1],c1);patch([0 1 1 1-e 1-e 0+e],[0 0 1 1-e 0+e 0+e],c2);patch([0 0 1 1-e 0+e 0+e],[0 1 1 1-e 1-e 0+e],c3);plot([0 1 1 0 0],[0 0 1 1 0]);
  wires:
  "IW{4,3}(1,:)'"/1 -> dotprod1/1
  "ad{4,3}"/1 -> dotprod1/2, dotprod2/2, dotprod3/2, dotprod4/2, dotprod5/2, dotprod6/2, dotprod7/2, dotprod8/2, dotprod9/2, dotprod10/2
  dotprod1/1 -> Mux/1
  "IW{4,3}(2,:)'"/1 -> dotprod2/1
  dotprod2/1 -> Mux/2
  "IW{4,3}(3,:)'"/1 -> dotprod3/1
  dotprod3/1 -> Mux/3
  "IW{4,3}(4,:)'"/1 -> dotprod4/1
  dotprod4/1 -> Mux/4
  "IW{4,3}(5,:)'"/1 -> dotprod5/1
  dotprod5/1 -> Mux/5
  "IW{4,3}(6,:)'"/1 -> dotprod6/1
  dotprod6/1 -> Mux/6
  "IW{4,3}(7,:)'"/1 -> dotprod7/1
  dotprod7/1 -> Mux/7
  "IW{4,3}(8,:)'"/1 -> dotprod8/1
  dotprod8/1 -> Mux/8
  "IW{4,3}(9,:)'"/1 -> dotprod9/1
  dotprod9/1 -> Mux/9
  "IW{4,3}(10,:)'"/1 -> dotprod10/1
  dotprod10/1 -> Mux/10
  Mux/1 -> "lz{4,3}"/1

== system nn_fuel_control_4_10/Air Fuel Control Model 1/Feed-Forward Neural Network1/Layer 5/Delays 1 ==
  "p{5}" : Inport  PortDimensions=10
      mask Display: e = 0.06;c1 = [120 230 180]/255;c2 = ([120 230 180]+0)/(256+128);c3 = ([120 230 180]+128)/(256+128);patch([0 1 1 0],[0 0 1 1],c1);patch([0 1 1 1-e 1-e 0+e],[0 0 1 1-e 0+e 0+e],c2);patch([0 0 1 1-e 0+e 0+e],[0 1 1 1-e 1-e 0+e],c3);plot([0 1 1 0 0],[0 0 1 1 0]);
  mux : Mux  Inputs=1
      mask Display: e = 0.06;c1 = [120 150 230]/255;c2 = ([120 150 230]+0)/383;c3 = ([120 150 230]+128)/383;patch([0 1 1 0],[0 0 1 1],c1);patch([0 1 1 1-e 1-e 0+e],[0 0 1 1-e 0+e 0+e],c2);patch([0 0 1 1-e 0+e 0+e],[0 1 1 1-e 1-e 0+e],c3);plot([0 1 1 0 0],[0 0 1 1 0]);disp('Mux')
  "pd{5,4}" : Outport
      mask Display: e = 0.06;c1 = [120 230 180]/255;c2 = ([120 230 180]+0)/(256+128);c3 = ([120 230 180]+128)/(256+128);patch([0 1 1 0],[0 0 1 1],c1);patch([0 1 1 1-e 1-e 0+e],[0 0 1 1-e 0+e 0+e],c2);patch([0 0 1 1-e 0+e 0+e],[0 1 1 1-e 1-e 0+e],c3);plot([0 1 1 0 0],[0 0 1 1 0]);
  wires:
  "p{5}"/1 -> mux/1
  mux/1 -> "pd{5,4}"/1

== system nn_fuel_control_4_10/Air Fuel Control Model 1/Feed-Forward Neural Network1/Layer 5/LW{5,4} ==
  "ad{5,4}" : Inport  PortDimensions=10
      mask Display: e = 0.06;c1 = [120 230 180]/255;c2 = ([120 230 180]+0)/(256+128);c3 = ([120 230 180]+128)/(256+128);patch([0 1 1 0],[0 0 1 1],c1);patch([0 1 1 1-e 1-e 0+e],[0 0 1 1-e 0+e 0+e],c2);patch([0 0 1 1-e 0+e 0+e],[0 1 1 1-e 1-e 0+e],c3);plot([0 1 1 0 0],[0 0 1 1 0]);
  "IW{5,4}(1,:)'" : Constant  Value=[-0.1673575207279787424585748567551490850746631622314453125;-0.0402600892327790449432001196328201331198215484619140625;0.378253528688959672621194840758107602596282958984375;0.7492896506042108217826580585096962749958038330078125;-0.2102870758909945181347467269006301648914813995361328125;-0.8548144420891092831737978485762141644954681396484375;0.334815016019122335677593582659028470516204833984375;0.7186319526555016157232103068963624536991119384765625;-0.49933573734407377120447790730395354330539703369140625;-0.12401842676148344679631918552331626415252685546875]
      mask Display: e = 0.06;c1 = [120 150 230]/255;c2 = ([120 150 230]+0)/383;c3 = ([120 150 230]+128)/383;patch([0 1 1 0],[0 0 1 1],c1);patch([0 1 1 1-e 1-e 0+e],[0 0 1 1-e 0+e 0+e],c2);patch([0 0 1 1-e 0+e 0+e],[0 1 1 1-e 1-e 0+e],c3);plot([0 1 1 0 0],[0 0 1 1 0]);disp('weights');
  Mux : Mux  Inputs=1
      mask Display: e = 0.06;c1 = [120 150 230]/255;c2 = ([120 150 230]+0)/383;c3 = ([120 150 230]+128)/383;patch([0 1 1 0],[0 0 1 1],c1);patch([0 1 1 1-e 1-e 0+e],[0 0 1 1-e 0+e 0+e],c2);patch([0 0 1 1-e 0+e 0+e],[0 1 1 1-e 1-e 0+e],c3);plot([0 1 1 0 0],[0 0 1 1 0]);disp('Mux');
  dotprod1 : neural/Weight Functions/dotprod
  "lz{5,4}" : Outport
      mask Display: e = 0.06;c1 = [120 230 180]/255;c2 = ([120 230 180]+0)/(256+128);c3 = ([120 230 180]+128)/(256+128);patch([0 1 1 0],[0 0 1 1],c1);patch([0 1 1 1-e 1-e 0+e],[0 0 1 1-e 0+e 0+e],c2);patch([0 0 1 1-e 0+e 0+e],[0 1 1 1-e 1-e 0+e],c3);plot([0 1 1 0 0],[0 0 1 1 0]);
  wires:
  "IW{5,4}(1,:)'"/1 -> dotprod1/1
  "ad{5,4}"/1 -> dotprod1/2
  dotprod1/1 -> Mux/1
  Mux/1 -> "lz{5,4}"/1
